simulink library "flightController_cl"  (R2020a)
settings: Solver=VariableStepAuto  StartTime=0.0  StopTime=10.0  RelTol=1e-3
libraries: calcBankAngle_cl x1, calcTangentRollAngle_ul x1, filteredPIDController_ul x1
settings Model: Creator=Ayaz  LastModifiedBy=Ayaz

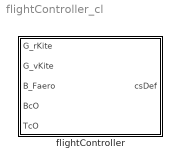
== system flightController_cl ==
  flightController : Subsystem  mask{PW=60, PH=28, PE=30, L1=0.05, initialPathParam=0, kiteMass=36.8, kp=1, ki=0, kd=0, tau=0.1}
      mask prompts: PW "Path width [deg]"; PH "Path height [deg]"; PE "Path mean elevation [deg]"; L1 "Normalized target forward length"; initialPathParam "Initial path parameter [rad]"; kiteMass "Kite mass [kg]"; kp "Proportional Gain, kp [rad/rad]"; ki "Integral Gain, ki [rad/rad*s]"; kd "Derivative Gain, kd [rad/rad/s]"; tau "Time Constant, s [s]"
      mask TypeOptions PW: calculateBankAngle/PW
      mask TypeOptions PH: calculateBankAngle/PH
      mask TypeOptions PE: calculateBankAngle/PE
      mask TypeOptions L1: calculateBankAngle/L1
      mask TypeOptions initialPathParam: calculateBankAngle/initialPathParam
      mask TypeOptions kiteMass: calculateBankAngle/kiteMass
      mask TypeOptions kp: filteredPIDController/kp
      mask TypeOptions ki: filteredPIDController/ki
      mask TypeOptions kd: filteredPIDController/kd
      mask TypeOptions tau: filteredPIDController/tau
      mask DialogControl Container3 Prompt: Airleron controller

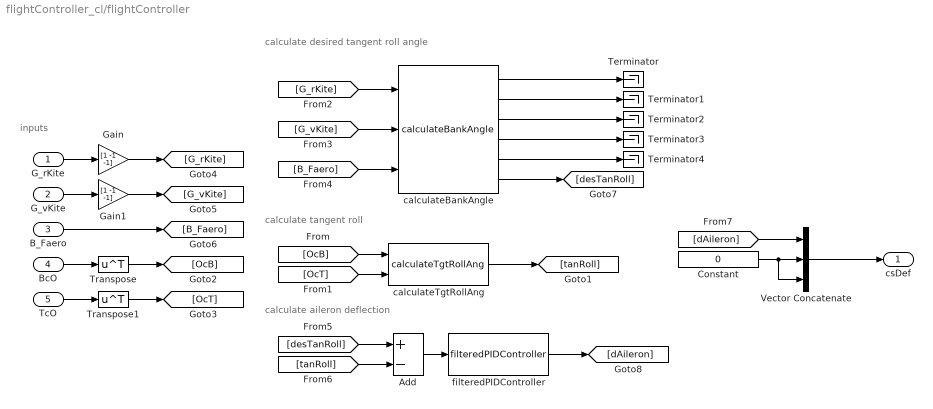
== system flightController_cl/flightController ==
  note: inputs
  note: calculate desired tangent roll angle
  note: calculate tangent roll
  note: calculate aileron deflection
  G_rKite : Inport
  G_vKite : Inport  Port=2
  B_Faero : Inport  Port=3
  BcO : Inport  Port=4
  TcO : Inport  Port=5
  Add : Sum  Inputs=+-
  Constant : Constant  Value=0
  Gain : Gain  Gain=[1 -1 -1]
  Gain1 : Gain  Gain=[1 -1 -1]
  Terminator{,1..4} (5 alike) : Terminator
  Transpose : Math  Operator=transpose  SaturateOnIntegerOverflow=on
  Transpose1 : Math  Operator=transpose  SaturateOnIntegerOverflow=on
  Vector Concatenate : Concatenate  NumInputs=3
  calculateBankAngle : calcBankAngle_cl/calculateBankAngle  PW=PW  PH=PH  PE=PE  L1=L1  initialPathParam=initialPathParam  kiteMass=kiteMass
  calculateTgtRollAng : calcTangentRollAngle_ul/calculateTgtRollAng  SystemSampleTime=-1  Latency=0  AutoFrameSizeCalculation=off
  filteredPIDController : filteredPIDController_ul/filteredPIDController  kp=kp  ki=ki  kd=kd  tau=tau  externalReset=none
  csDef : Outport
  wires:
  [OcB] -> calculateTgtRollAng/1
  [OcT] -> calculateTgtRollAng/2
  calculateTgtRollAng/1 -> [tanRoll]
  [G_rKite] -> calculateBankAngle/1
  [G_vKite] -> calculateBankAngle/2
  [B_Faero] -> calculateBankAngle/3
  calculateBankAngle/6 -> [desTanRoll]
  [desTanRoll] -> Add/1
  [tanRoll] -> Add/2
  Add/1 -> filteredPIDController/1
  filteredPIDController/1 -> [dAileron]
  [dAileron] -> Vector Concatenate/1
  Constant/1 -> Vector Concatenate/3, Vector Concatenate/2
  Vector Concatenate/1 -> csDef/1
  calculateBankAngle/1 -> Terminator/1
  calculateBankAngle/2 -> Terminator1/1
  calculateBankAngle/3 -> Terminator2/1
  calculateBankAngle/4 -> Terminator3/1
  calculateBankAngle/5 -> Terminator4/1
  G_rKite/1 -> Gain/1
  G_vKite/1 -> Gain1/1
  B_Faero/1 -> [B_Faero]
  BcO/1 -> Transpose/1
  Transpose/1 -> [OcB]
  TcO/1 -> Transpose1/1
  Transpose1/1 -> [OcT]
  Gain/1 -> [G_rKite]
  Gain1/1 -> [G_vKite]
